simulink model "SU_demo"  (R2023b)
settings: Solver=FixedStepDiscrete  StartTime=0.0  StopTime=130  FixedStep=1/2400  RelTol=1e-3  EnableMultiTasking=on
model workspace (MAT data in the model file):
  buffer_size = 16
  cfg_native : object (value not decoded)
  device_serial = 'HA-2016.09.02'
  number_of_channels = 7
  sample_rate = 2400
undefined symbols (not defined in the file or in its folder): ES, PULSE, SR, TRAIN
libraries: simulink x4, Visualization x2, DataStream x1, SwitchingUnitSimulinkLibrary x1, gEstimPRO x1, DataAcquisition x1
settings Model: ModifiedByFormat=g.tec  Creator=HalpernLab.NK  LastModifiedBy=g.tec
settings SolverCC: AlgebraicLoopSolver=TrustRegion  AutoInsertRateTranBlk=on
settings DataIOCC: LimitDataPoints=on  SaveFormat=Array  ReturnWorkspaceOutputs=off
settings OptimizationCC: LifeSpan=inf
settings DebuggingCC: UnconnectedInputMsg=warning  UnconnectedOutputMsg=warning  UnconnectedLineMsg=warning  SFUnexpectedBacktrackingDiag=warning  SFNoUnconditionalDefaultTransitionDiag=warning  SFExecutionAtInitializationDiag=none  ArithmeticOperatorsInVariantConditions=warning
settings HardwareCC: ProdBitPerPointer=32  ProdBitPerSizeT=32  ProdBitPerPtrDiffT=32  ProdLargestAtomicFloat=None  ProdIntDivRoundTo=Undefined  ProdEndianess=Unspecified  ProdWordSize=32  ProdHWDeviceType=32-bit Generic
settings ModelReferenceCC: EnableRefExpFcnMdlSchedulingChecks=on  PropagateSignalLabelsOutOfModel=off
settings SFSimCC: SimUseLocalCustomCode=off  CustomCodeUndefinedFunction=UseInterfaceOnly
settings RTWCC: RTWUseLocalCustomCode=off
settings CodeAppCC: StateflowObjectComments=on
settings GRTTargetCC: TargetLangStandard=C89/C90 (ANSI)
settings ConfigComp: CovMetricSettings=dw  CovSaveCumulativeToWorkspaceVar=on  CovSaveSingleToWorkspaceVar=on  CovExternalEMLEnable=off

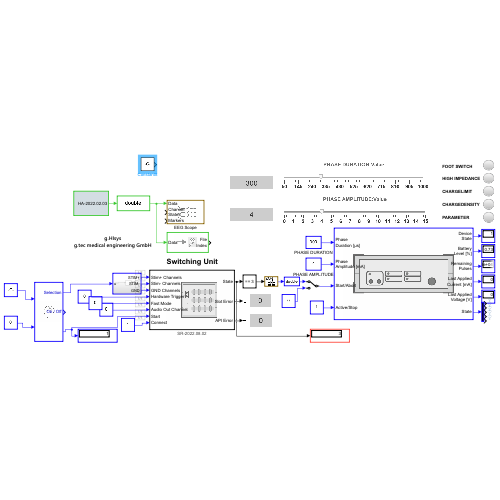
[thumbnail: Simulink's stored preview of the top-level diagram]
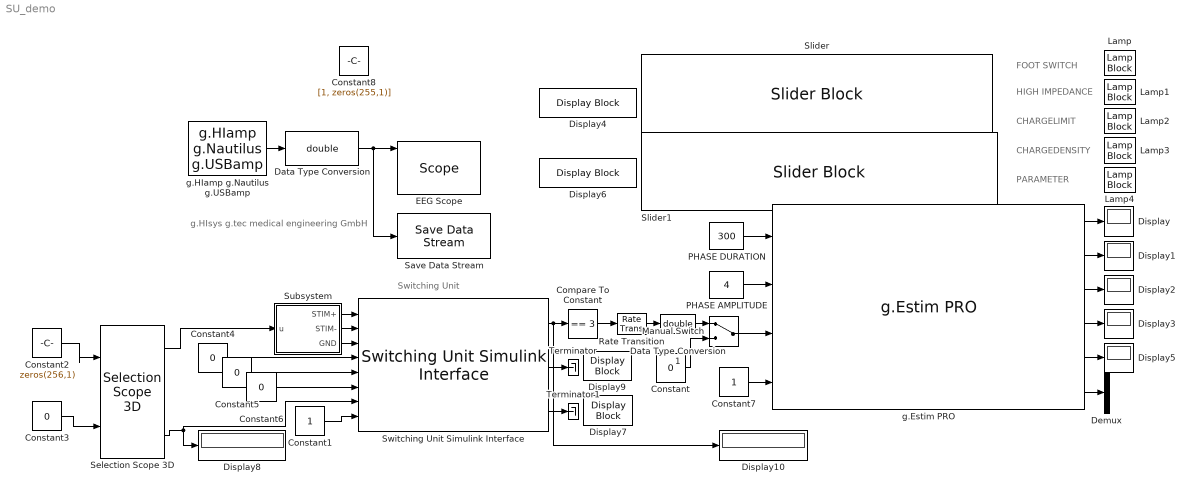
== system SU_demo ==
  note: Switching Unit
  note: g.HIsys
      | g.tec medical engineering GmbH
  note: HIGH IMPEDANCE
  note: CHARGEDENSITY
  note: CHARGELIMIT
  note: FOOT SWITCH
  note: PARAMETER
  Compare To Constant : simulink/Logic and Bit Operations/Compare To Constant  relop===  const=3  OutDataTypeStr=boolean
  Constant : Constant  Value=0  SampleTime=1/150
  Constant1 : Constant  SampleTime=1/100
  Constant2 : Constant  Value=zeros(256,1)  SampleTime=1/100
  Constant3 : Constant  Value=0  SampleTime=1/100
  Constant4 : Constant  Value=0  SampleTime=1/100
  Constant5 : Constant  Value=0  SampleTime=1/100
  Constant6 : Constant  Value=0  SampleTime=1/150
  Constant7 : Constant  SampleTime=1/150
  Constant8 : Constant  Value=[1, zeros(255,1)]
  Data Type Conversion : DataTypeConversion  OutDataTypeStr=double  SaturateOnIntegerOverflow=off  RndMeth=Floor
  Data Type Conversion1 : DataTypeConversion  OutDataTypeStr=double  SaturateOnIntegerOverflow=off  RndMeth=Floor
  Demux : Demux  Outputs=5
  Display{,1..3,5,8,10} (7 alike) : Display
  Display4 : DisplayBlock  LabelPosition=Hide  Format=Integer  Transparency=1  FormatString=%i
  Display6 : DisplayBlock  LabelPosition=Hide  Transparency=1
  Display7 : DisplayBlock  LabelPosition=Hide  Format=Integer  Transparency=1  FormatString=%i
  Display9 : DisplayBlock  LabelPosition=Hide  Format=Integer  Transparency=1  FormatString=%i
  EEG Scope : Visualization/Scope
      settings: SourceProductName=g.HIsys
  Lamp{,1..4} (5 alike) : LampBlock  LabelPosition=Hide
  Manual Switch : ManualSwitch
  PHASE AMPLITUDE : Constant  Value=4  SampleTime=1/150
  PHASE DURATION : Constant  Value=300  SampleTime=1/150
  Rate Transition : RateTransition  OutPortSampleTime=1/150
  Save Data Stream : DataStream/Save Data Stream  filename=file.mat  filesize=1024  blocksize=1  rec_type=Single  enable=off  save_model=off  save_pp_taskinfo=off  patient_data=off  id=ID0000  firstname=John  lastname=Doe  dateofbirth=12.01.2001  sex=MALE  hand=RIGHT  diagnosis=Diagnosis  medication=Medication Text  comments=any text ...  run=1  session=1
      settings: SourceProductName=g.HIsys
  Selection Scope 3D : Visualization/Selection Scope 3D  defaultConfigPath=''
      settings: SourceProductName=g.HIsys
  Slider : SliderBlock  ScaleMin=50  ScaleMax=1000
  Slider1 : SliderBlock  ScaleMax=15
  Subsystem : Subsystem
  Switching Unit Simulink Interface : SwitchingUnitSimulinkLibrary/Switching Unit Simulink Interface  dev_idx=0  snr=SR-2022.08.02
      settings: AttributesFormatString=SR-2022.08.02  SourceProductName=g.HIsys
  Terminator : Terminator
  Terminator1 : Terminator
  g.Estim PRO : gEstimPRO/g.Estim PRO  serial=ES-2020.04.02  old_serial=ES-2020.04.02  supermode_enabled=off  DI1_enabled=off  buzzer_enabled=on  surface_area_mm2=4  interphase_time=0  modality=BIPHASIC  polarity=ALTERNATING  pulses=13000  pulse_rate=130  fade_type=BOTH  fade_in_time=0  fade_out_time=0  digout1_mode=1 - TRAIN  digout1_pre=0  digout1_post=0  digout2_mode=2 - PULSE  digout2_pre=0  digout2_post=0
      settings: SourceProductName=g.HIsys
  g.HIamp g.Nautilus g.USBamp : DataAcquisition/g.HIamp g.Nautilus g.USBamp  cfgUpdated=739499.3982  numDevices=2  deviceSR=[500 250 ]  deviceChannels=[9 4 ]  numSR=[2 ]  SRIndexPerDevice=[1 0 ]
      settings: SourceProductName=g.HIsys
  wires:
  Data Type Conversion/1 -> Save Data Stream/1, EEG Scope/1
  g.HIamp g.Nautilus g.USBamp/1 -> Data Type Conversion/1
  g.Estim PRO/1 -> Display/1
  g.Estim PRO/2 -> Display1/1
  Constant/1 -> Manual Switch/2
  Switching Unit Simulink Interface/1 -> Display10/1, Compare To Constant/1
  g.Estim PRO/5 -> Display5/1
  g.Estim PRO/6 -> Demux/1
  g.Estim PRO/4 -> Display3/1
  g.Estim PRO/3 -> Display2/1
  Data Type Conversion1/1 -> Manual Switch/1
  Manual Switch/1 -> g.Estim PRO/3
  PHASE AMPLITUDE/1 -> g.Estim PRO/2
  PHASE DURATION/1 -> g.Estim PRO/1
  Switching Unit Simulink Interface/2 -> Terminator/1
  Switching Unit Simulink Interface/3 -> Terminator1/1
  Subsystem/1(STIM+) -> Switching Unit Simulink Interface/1
  Subsystem/2(STIM-) -> Switching Unit Simulink Interface/2
  Subsystem/3(GND) -> Switching Unit Simulink Interface/3
  Constant1/1 -> Switching Unit Simulink Interface/8
  Constant2/1 -> Selection Scope 3D/1
  Compare To Constant/1 -> Rate Transition/1
  Rate Transition/1 -> Data Type Conversion1/1
  Constant3/1 -> Selection Scope 3D/2
  Selection Scope 3D/1 -> Subsystem/1(u)
  Constant4/1 -> Switching Unit Simulink Interface/4
  Constant5/1 -> Switching Unit Simulink Interface/5
  Constant6/1 -> Switching Unit Simulink Interface/6
  Selection Scope 3D/3 -> Switching Unit Simulink Interface/7, Display8/1
  Constant7/1 -> g.Estim PRO/4

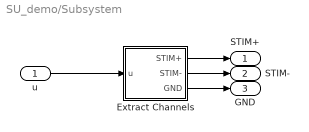
== system SU_demo/Subsystem ==
  u : Inport
  Extract Channels : Subsystem
  STIM+ : Outport
  STIM- : Outport  Port=2
  GND : Outport  Port=3
  wires:
  u/1 -> Extract Channels/1(u)
  Extract Channels/1(STIM+) -> STIM+/1
  Extract Channels/3(GND) -> GND/1
  Extract Channels/2(STIM-) -> STIM-/1

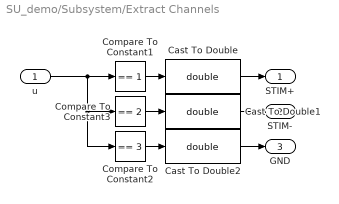
== system SU_demo/Subsystem/Extract Channels ==
  u : Inport
  Cast To Double : DataTypeConversion  OutDataTypeStr=double  SaturateOnIntegerOverflow=off  RndMeth=Floor
  Cast To Double1 : DataTypeConversion  OutDataTypeStr=double  SaturateOnIntegerOverflow=off  RndMeth=Floor
  Cast To Double2 : DataTypeConversion  OutDataTypeStr=double  SaturateOnIntegerOverflow=off  RndMeth=Floor
  Compare To Constant1 : simulink/Logic and Bit Operations/Compare To Constant  relop===  const=1  OutDataTypeStr=boolean
  Compare To Constant2 : simulink/Logic and Bit Operations/Compare To Constant  relop===  const=3  OutDataTypeStr=boolean
  Compare To Constant3 : simulink/Logic and Bit Operations/Compare To Constant  relop===  const=2  OutDataTypeStr=boolean
  STIM+ : Outport
  STIM- : Outport  Port=2
  GND : Outport  Port=3
  wires:
  u/1 -> Compare To Constant1/1, Compare To Constant2/1, Compare To Constant3/1
  Compare To Constant3/1 -> Cast To Double1/1
  Cast To Double2/1 -> GND/1
  Compare To Constant2/1 -> Cast To Double2/1
  Cast To Double/1 -> STIM+/1
  Compare To Constant1/1 -> Cast To Double/1
  Cast To Double1/1 -> STIM-/1
